simulink model "lab2_2"  (R2016a)
settings: Solver=ode1  StartTime=0.0  StopTime=100  FixedStep=0.01  RelTol=1e-3
settings Model: Creator=ms36124  LastModifiedBy=ms36124

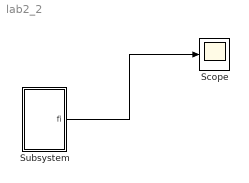
== system lab2_2 ==
  Scope : Scope
  Subsystem : Subsystem  mask{m=10, k=1, l=3, g=10, fi0=90}
  wires:
  Subsystem/1("fi ") -> Scope/1

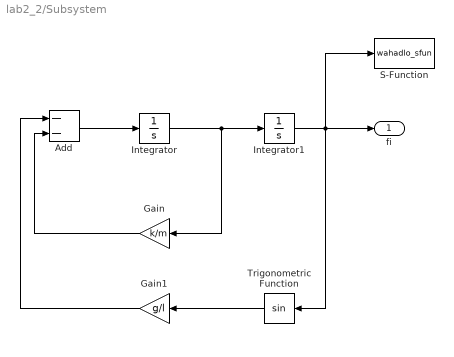
== system lab2_2/Subsystem ==
  Add : Sum  Inputs=--
  Gain : Gain  Gain=k/m
  Gain1 : Gain  Gain=g/l
  Integrator : Integrator
  Integrator1 : Integrator  InitialCondition=fi0*pi/180
  S-Function : S-Function  FunctionName=wahadlo_sfun  Parameters=l,m,fi0  SFunctionDeploymentMode=off  EnableBusSupport=off
  Trigonometric Function : Trigonometry
  "fi " : Outport
  wires:
  Trigonometric Function/1 -> Gain1/1
  Integrator/1 -> Gain/1, Integrator1/1
  Add/1 -> Integrator/1
  Integrator1/1 -> S-Function/1, "fi "/1, Trigonometric Function/1
  Gain1/1 -> Add/1
  Gain/1 -> Add/2
